simulink model "Workshop_0_43"  (R2019b)
settings: Solver=VariableStepAuto  StartTime=0.0  StopTime=10.0  RelTol=1e-3
settings Model: Creator=linesLK  LastModifiedBy=linesLK

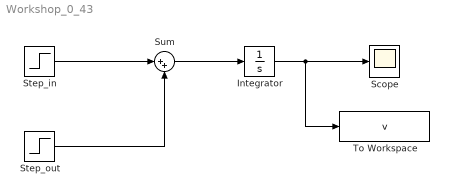
== system Workshop_0_43 ==
  Integrator : Integrator
  Scope : Scope
  Step_in : Step  SampleTime=0
  Step_out : Step  SampleTime=0
  Sum : Sum  Inputs=|++
  To Workspace : ToWorkspace  VariableName=v  SaveFormat=Timeseries  SampleTime=-1
  wires:
  Step_in/1 -> Sum/1
  Step_out/1 -> Sum/2
  Sum/1 -> Integrator/1
  Integrator/1 -> To Workspace/1, Scope/1
